simulink model "Group44AOO"  (R2022b)
settings: Solver=FixedStepAuto  StartTime=0.0  StopTime=10.0  FixedStep=1e-3  RelTol=1e-3  EnableMultiTasking=on
undefined symbols (not defined in the file): D10, D11, D12, D2, D4, D5, D7, D8, D9, PTA0, PTA2, PTB23, PTB9, PTC3, PTC4, PTD0, PTD2, PTD3
libraries: frdmk64flib x9
settings Model: ExtModeTrigDuration=5  Creator=Admin  LastModifiedBy=Admin
settings OptimizationCC: EnhancedBackFolding=on  PassReuseOutputArgsAs=Individual arguments  ZeroExternalMemoryAtStartup=off  ZeroInternalMemoryAtStartup=off  MaxStackSize=64  OptimizeBlockOrder=speed  DifferentSizesBufferReuse=on  OptimizationCustomize=off  EfficientTunableParamExpr=on
settings DebuggingCC: ParameterTunabilityLossMsg=error
settings HardwareCC: ProdBitPerPointer=32  ProdBitPerSizeT=32  ProdBitPerPtrDiffT=32  ProdLargestAtomicInteger=Long  ProdLargestAtomicFloat=Double  ProdWordSize=32  ProdHWDeviceType=ARM Compatible->ARM Cortex
settings SFSimCC: MATLABDynamicMemAlloc=off
settings RTWCC: Description=Embedded Coder  SystemTargetFile=ert.tlc  HardwareBoard=NXP FRDM-K64F  TLCOptions="-aInlineSetEventsForThisBaseRateFcn=TLC_FALSE -aSuppressMultiTaskScheduler=TLC_FALSE  -aRateBasedStepFcn=0"  TemplateMakefile=ert_default_tmf  Toolchain=GNU Tools for ARM Embedded Processors
settings CodeAppCC: ForceParamTrailComments=on  IgnoreCustomStorageClasses=off  OperatorAnnotations=on  SimulinkDataObjDesc=on  SFDataObjDesc=on  InsertBlockDesc=on
settings ERTTargetCC: ExtModeTransport=4  ExtModeMexFile=sendToCommService

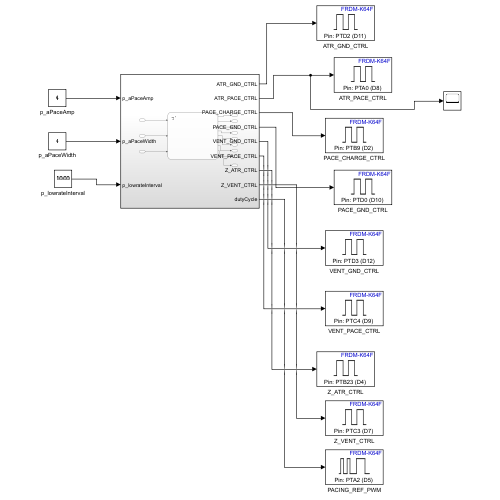
[thumbnail: Simulink's stored preview of the top-level diagram]
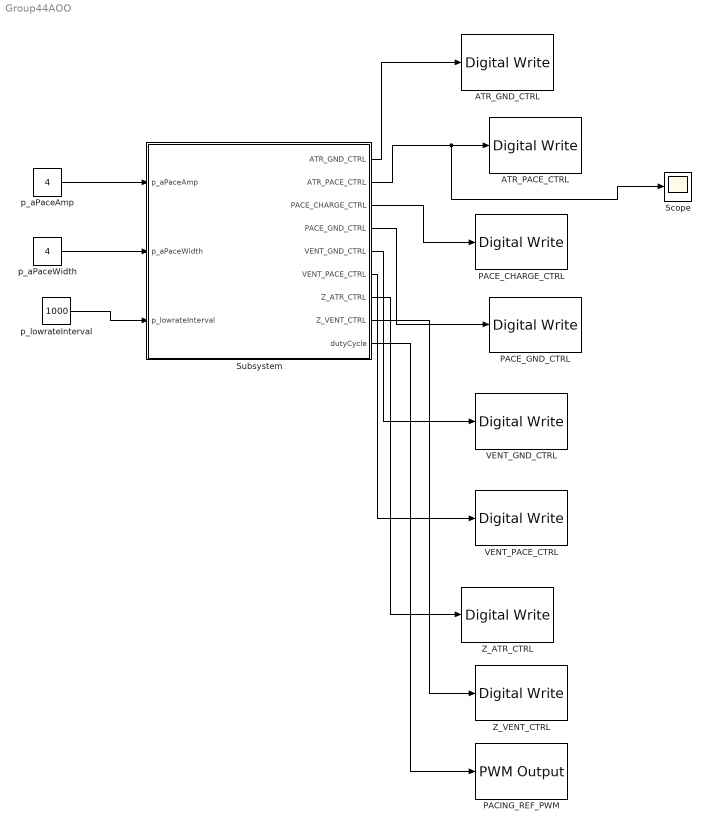
== system Group44AOO ==
  ATR_GND_CTRL : frdmk64flib/Digital Write  Whichpin=PTD2 (D11)
  ATR_PACE_CTRL : frdmk64flib/Digital Write  Whichpin=PTA0 (D8)
  PACE_CHARGE_CTRL : frdmk64flib/Digital Write  Whichpin=PTB9 (D2)
  PACE_GND_CTRL : frdmk64flib/Digital Write  Whichpin=PTD0 (D10)
  PACING_REF_PWM : frdmk64flib/PWM Output  Whichpin=PTA2 (D5)  InitialFrequency=2000  InitialDutyCycle=0
  Scope : Scope
  Subsystem : Subsystem
  VENT_GND_CTRL : frdmk64flib/Digital Write  Whichpin=PTD3 (D12)
  VENT_PACE_CTRL : frdmk64flib/Digital Write  Whichpin=PTC4 (D9)
  Z_ATR_CTRL : frdmk64flib/Digital Write  Whichpin=PTB23 (D4)
  Z_VENT_CTRL : frdmk64flib/Digital Write  Whichpin=PTC3 (D7)
  p_aPaceAmp : Constant  Value=4  OutDataTypeStr=double
  p_aPaceWidth : Constant  Value=4  OutDataTypeStr=double
  p_lowrateInterval : Constant  Value=1000  OutDataTypeStr=double
  wires:
  Subsystem/1(ATR_GND_CTRL) -> ATR_GND_CTRL/1
  Subsystem/2(ATR_PACE_CTRL) -> Scope/1, ATR_PACE_CTRL/1
  Subsystem/3(PACE_CHARGE_CTRL) -> PACE_CHARGE_CTRL/1
  Subsystem/4(PACE_GND_CTRL) -> PACE_GND_CTRL/1
  Subsystem/5(VENT_GND_CTRL) -> VENT_GND_CTRL/1
  Subsystem/6(VENT_PACE_CTRL) -> VENT_PACE_CTRL/1
  Subsystem/7(Z_ATR_CTRL) -> Z_ATR_CTRL/1
  Subsystem/8(Z_VENT_CTRL) -> Z_VENT_CTRL/1
  p_aPaceWidth/1 -> Subsystem/2(p_aPaceWidth)
  p_lowrateInterval/1 -> Subsystem/3(p_lowrateInterval)
  Subsystem/9(dutyCycle) -> PACING_REF_PWM/1
  p_aPaceAmp/1 -> Subsystem/1(p_aPaceAmp)

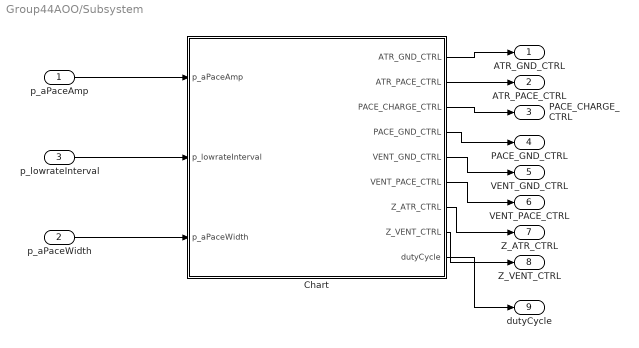
== system Group44AOO/Subsystem ==
  p_aPaceAmp : Inport
  p_aPaceWidth : Inport  Port=2
  p_lowrateInterval : Inport  Port=3
  Chart : Stateflow chart  TreatAsAtomicUnit=on
      settings: PortSchema="{\"entries\":[{\"content\":{\"sides\":[{\"content\":{\"connectorIds\":[\"In3\",\"In2\",\"In1\"]},\"type\":\"ConnectorPlacement.EquallySpacedRectSide\",\"uuid\":\"f4dc3048-51d6-4db6-b265-a066d0dfda2d\"},{\"content\":{\"connectorIds\":[\"Out1\",\"Out2\",\"Out3\",\"Out4\",\"Out5\",\"Out6\",\"Out7\",\"Out8\",\"Out9\"],\"side\":\"RIGHT\"},\"type\":\"ConnectorPlacement.EquallySpacedRectSide\",\"uuid\":\"825f81e3-5cfe-4fd7-b9fc-d4806473552a\"},{\"content\":{\"connectorIds\":[],\"side\":\"TOP\"},\"type\":\"ConnectorPlacement.EquallySpacedRectSide\",\"uuid\":\"498485ba-e1f2-445a-9610-e3b27215c6f8\"}]},\"type\":\"ConnectorPlacement.EquallySpacedConnector\",\"uuid\":\"f957d02a-744b-46bb-8823-515c8e1b2a98\"}],\"packageUris\":[\"http://schema.mathworks.com/mf0/Connector/R2020b\"],\"version\":\"1.0\"}"
  ATR_GND_CTRL : Outport
  ATR_PACE_CTRL : Outport  Port=2
  PACE_CHARGE_CTRL : Outport  Port=3
  PACE_GND_CTRL : Outport  Port=4
  VENT_GND_CTRL : Outport  Port=5
  VENT_PACE_CTRL : Outport  Port=6
  Z_ATR_CTRL : Outport  Port=7
  Z_VENT_CTRL : Outport  Port=8
  dutyCycle : Outport  Port=9
  wires:
  p_aPaceAmp/1 -> Chart/3(p_aPaceAmp)
  Chart/1(ATR_GND_CTRL) -> ATR_GND_CTRL/1
  Chart/2(ATR_PACE_CTRL) -> ATR_PACE_CTRL/1
  Chart/3(PACE_CHARGE_CTRL) -> PACE_CHARGE_CTRL/1
  Chart/4(PACE_GND_CTRL) -> PACE_GND_CTRL/1
  Chart/5(VENT_GND_CTRL) -> VENT_GND_CTRL/1
  Chart/6(VENT_PACE_CTRL) -> VENT_PACE_CTRL/1
  Chart/7(Z_ATR_CTRL) -> Z_ATR_CTRL/1
  Chart/8(Z_VENT_CTRL) -> Z_VENT_CTRL/1
  Chart/9(dutyCycle) -> dutyCycle/1
  p_lowrateInterval/1 -> Chart/2(p_lowrateInterval)
  p_aPaceWidth/1 -> Chart/1(p_aPaceWidth)

== stateflow chart Group44AOO/Subsystem/Chart ==
  state ChargeC22_Atrial_DischargeC21
    entry:
    ATR_PACE_CTRL = false;
    VENT_PACE_CTRL = false;
    PACE_CHARGE_CTRL = true;
    PACE_GND_CTRL = true;
    Z_ATR_CTRL = false;
    Z_VENT_CTRL = false;
    ATR_GND_CTRL = true;
    VENT_GND_CTRL = false;
    dutyCycle=p_aPaceAmp/5.0*100
  state PaceAtria
    entry:
    PACE_CHARGE_CTRL = false;
    PACE_GND_CTRL = true;
    ATR_PACE_CTRL = true;
    ATR_GND_CTRL = false;
    Z_ATR_CTRL = false;
    Z_VENT_CTRL = false;
    VENT_GND_CTRL = false;
    VENT_PACE_CTRL = false;
    %natPaceDetected=false;
  (default) -> ChargeC22_Atrial_DischargeC21
  ChargeC22_Atrial_DischargeC21 -> PaceAtria : after(p_lowrateInterval-p_aPaceWidth,msec)
  PaceAtria -> ChargeC22_Atrial_DischargeC21 : after(p_aPaceWidth,msec)
  data: p_aPaceWidth input; p_lowrateInterval input; ATR_GND_CTRL output; ATR_PACE_CTRL output; PACE_CHARGE_CTRL output; PACE_GND_CTRL output; VENT_GND_CTRL output; VENT_PACE_CTRL output; Z_ATR_CTRL output; Z_VENT_CTRL output; dutyCycle output; p_aPaceAmp input
